simulink model "UPDATED_2"  (R2025a)
settings: Solver=VariableStepAuto  StartTime=0.0  StopTime=0  RelTol=1e-3
libraries: spsPWMGeneratorDCDCLib x8, spsSeriesRLCBranchLib x6, spsCurrentMeasurementLib x5, spsMosfetLib x4, spsVoltageMeasurementLib x3, eeStairGenerator x2, spsDCVoltageSourceLib x1, spsGroundLib x1, sps_lib x1
settings Model: Creator=KAILASH  LastModifiedBy=KAILASH

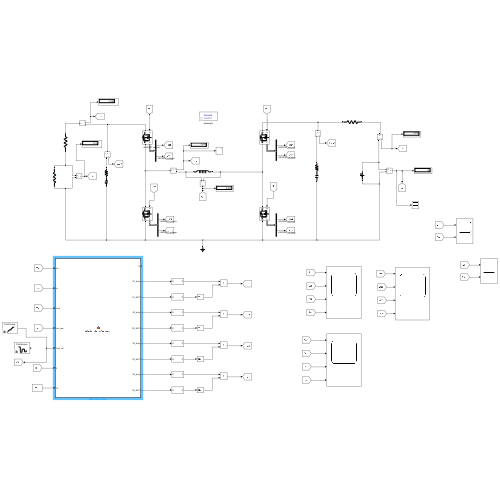
[thumbnail: Simulink's stored preview of the top-level diagram]
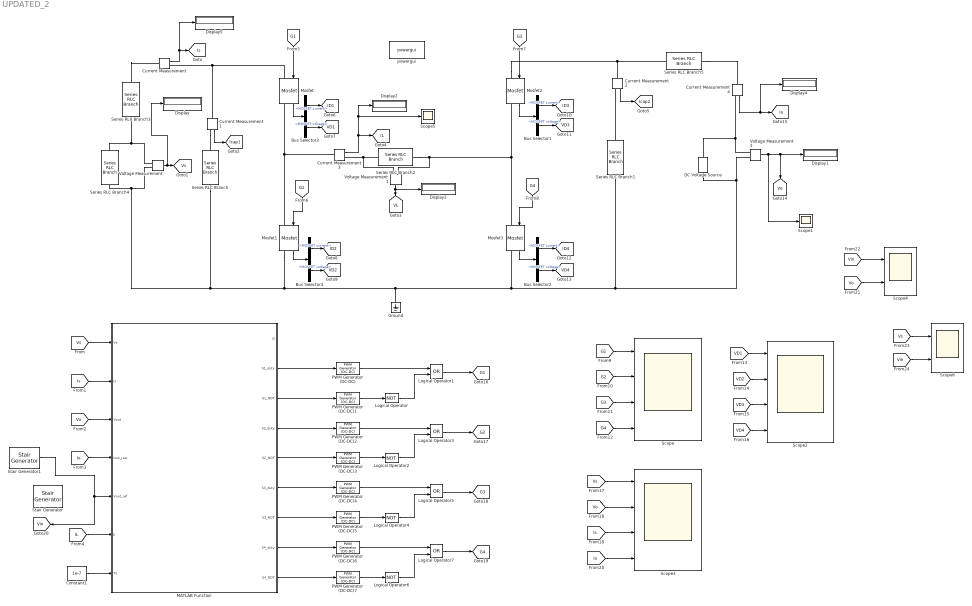
== system UPDATED_2 ==
  Bus Selector{1..4} (4 alike) : BusSelector  OutputSignals=MOSFET current,MOSFET voltage
  Constant1 : Constant  Value=1e-7
  Current Measurement{,1..4} (5 alike) : spsCurrentMeasurementLib/Current Measurement  PhasorSimulation=off  OutputType=Complex  PSBequivalent=0
  DC Voltage Source : spsDCVoltageSourceLib/DC Voltage Source  Amplitude=48  Measurements=Voltage
  Display{,1..5} (6 alike) : Display
  Ground : spsGroundLib/Ground  LConnTagsString=a
  Logical Operator{,2,4,6} (4 alike) : Logic  Operator=NOT  AllPortsSameDT=off  OutDataTypeStr=boolean
  Logical Operator{1,3,5,7} (4 alike) : Logic  Operator=OR  AllPortsSameDT=off  OutDataTypeStr=boolean
  MATLAB Function : MATLAB Function  TreatAsAtomicUnit=on
  Mosfet{,1..3} (4 alike) : spsMosfetLib/Mosfet  Ron=0.01  Lon=0  Rd=0.01  Vfd=0.8  IC=0  Rs=1e5  Cs=inf  Measurements=on
  PWM Generator (DC-DC){,1..7} (8 alike) : spsPWMGeneratorDCDCLib/PWM Generator (DC-DC)  Fsw=75e3  Ts=1e-7
  Scope : Scope  NumInputPorts=4
      settings: ActiveDisplayYMinimum=0.9  ActiveDisplayYMaximum=1.1
  Scope1 : Scope
      settings: ActiveDisplayYMinimum=-5.735151236633631  ActiveDisplayYMaximum=51.67637083167557
  Scope2 : Scope  NumInputPorts=4
      settings: ActiveDisplayYMinimum=-4.0101855999563254  ActiveDisplayYMaximum=36.044750018114769  DataLoggingVariableName=ScopeData2
  Scope3 : Scope  NumInputPorts=4
      settings: ActiveDisplayYMinimum=38  ActiveDisplayYMaximum=58  DataLoggingVariableName=ScopeData3
  Scope4 : Scope  NumInputPorts=2
      settings: ActiveDisplayYMinimum=-8.760106786096161  ActiveDisplayYMaximum=78.7511229762329  DataLoggingVariableName=ScopeData4
  Scope5 : Scope
      settings: ActiveDisplayYMinimum=-12.405117620742399  ActiveDisplayYMaximum=103.6893246645467  DataLoggingVariableName=ScopeData5
  Scope6 : Scope  NumInputPorts=2
      settings: ActiveDisplayYMinimum=-11.293274527726584  ActiveDisplayYMaximum=84.8994228584227  DataLoggingVariableName=ScopeData6
  Series RLC Branch : spsSeriesRLCBranchLib/Series RLC Branch  LConnTagsString=__new0  RConnTagsString=__new0  BranchType=RC  Resistance=0.001  Inductance=1e-3  SetiL0=off  InitialCurrent=0  Capacitance=488e-6  Setx0=off  InitialVoltage=48  Measurements=None
  Series RLC Branch1 : spsSeriesRLCBranchLib/Series RLC Branch  LConnTagsString=__new0  RConnTagsString=__new0  BranchType=RC  Resistance=0.01  Inductance=1e-3  SetiL0=off  InitialCurrent=0  Capacitance=488e-6  Setx0=off  InitialVoltage=36  Measurements=None
  Series RLC Branch2 : spsSeriesRLCBranchLib/Series RLC Branch  LConnTagsString=__new0  RConnTagsString=__new0  BranchType=L  Resistance=1  Inductance=200e-6  SetiL0=off  InitialCurrent=0  Capacitance=1e-6  Setx0=off  InitialVoltage=0  Measurements=None
  Series RLC Branch3 : spsSeriesRLCBranchLib/Series RLC Branch  LConnTagsString=__new0  RConnTagsString=__new0  BranchType=R  Resistance=1  Inductance=1e-3  SetiL0=off  InitialCurrent=0  Capacitance=1e-6  Setx0=off  InitialVoltage=0  Measurements=None
  Series RLC Branch4 : spsSeriesRLCBranchLib/Series RLC Branch  LConnTagsString=__new0  RConnTagsString=__new0  BranchType=R  Resistance=50  Inductance=1e-3  SetiL0=off  InitialCurrent=0  Capacitance=1e-6  Setx0=off  InitialVoltage=0  Measurements=None
  Series RLC Branch5 : spsSeriesRLCBranchLib/Series RLC Branch  LConnTagsString=__new0  RConnTagsString=__new0  BranchType=R  Resistance=1  Inductance=1e-3  SetiL0=off  InitialCurrent=0  Capacitance=1e-6  Setx0=off  InitialVoltage=0  Measurements=None
  Stair Generator : eeStairGenerator/Stair Generator  LabelModeActiveChoice=Continuous  TimeInput=[0.05 0.2 0.35 0.55 0.7]  AmplitudeInput=[90 6 55 12 36]  SampleTime=0  RepeatPattern=off  OutDataTypeStr=double
      settings: LibrarySourceBlock=ee_sl_lib/General Control/Stair Generator
  Stair Generator1 : eeStairGenerator/Stair Generator  LabelModeActiveChoice=Continuous  TimeInput=[0.05 0.2 0.35 0.55 0.7 0.85]  AmplitudeInput=[52 64 70 82 90 92]  SampleTime=0  RepeatPattern=off  OutDataTypeStr=double
      settings: LibrarySourceBlock=ee_sl_lib/General Control/Stair Generator
  Voltage Measurement : spsVoltageMeasurementLib/Voltage Measurement  PhasorSimulation=off  OutputType=Complex  PSBequivalent=0
  Voltage Measurement1 : spsVoltageMeasurementLib/Voltage Measurement  PhasorSimulation=off  OutputType=Complex  PSBequivalent=0
  Voltage Measurement2 : spsVoltageMeasurementLib/Voltage Measurement  PhasorSimulation=off  OutputType=Complex  PSBequivalent=0
  powergui : sps_lib/powergui  Priority=1  SimulationMode=Discrete  SampleTime=1e-7  frequency=60  Iterations=50  frequencyindice=0  Pbase=100e6  ErrMax=1e-4  UnitsV=kV  UnitsW=MW  buscounter=0  FunctionMessages=off  echomessages=off  EnableUseOfTLC=off  CurrentSourceSwitches=off  DisableSnubberDevices=off  DisableRonSwitches=off  DisableVfSwitches=off  DisplayEquations=off  AutomaticDiscreteSolvers=off  SolverType=Tustin/Backward Euler (TBE)  Interpol=off  ExternalGateDelay=off  methode=off  Ts=100  x0status=blocks  SPID=on  SwTol=0  HookPort=off  NonlinearTolerance=1e-4  nMaxIteration=100  ContinueOnMaxIteration=off  RestoreLinks=warning  ResistiveCurrentMeasurement=off  Frange=[0:2:500]  Ylog=off  Xlog=on  ShowGrid=off  save=off  variable=ZData  structure=0  ZoomFFT=off  StartTime=0.0  cycles=1  DisplayStyle=1  fundamental=60  FreqAxis=off  MaxFrequency=1000  frequencyindicesteady=1  RmsSteady=1  display=off
  tag scope: G1=global, G2=global, G3=global, G4=global, ID1=global, ID2=global, ID3=global, ID4=global, IL=global, Icap1=global, Icap2=global, Io=global, Is=global, VD1=global, VD2=global, VD3=global, VD4=global, VL=global, Vin=global, Vo=global, Vs=global
  wires:
  MATLAB Function/5(S2_NOT) -> PWM Generator (DC-DC)3/1
  Current Measurement1/1 -> [Icap1]
  Mosfet/1 -> Bus Selector3/1
  Bus Selector2/1 -> [ID4]  "<MOSFET current>"
  [G1] -> Scope/1
  MATLAB Function/7(S3_NOT) -> PWM Generator (DC-DC)5/1
  [Is] -> MATLAB Function/2(Is)
  MATLAB Function/8(S4_duty) -> PWM Generator (DC-DC)6/1
  [VD3] -> Scope2/3
  [Vo] -> Scope4/2
  PWM Generator (DC-DC)1/1 -> Logical Operator/1
  MATLAB Function/2(S1_duty) -> PWM Generator (DC-DC)/1
  PWM Generator (DC-DC)7/1 -> Logical Operator6/1
  Current Measurement3/1 -> [IL], Scope5/1, Display2/1
  Constant1/1 -> MATLAB Function/7(Ts)
  [Vo] -> MATLAB Function/3(Vout)
  Logical Operator7/1 -> [G4]
  Current Measurement/1 -> Display5/1, [Is]
  Mosfet1/1 -> Bus Selector4/1
  Logical Operator2/1 -> Logical Operator3/2
  [VD4] -> Scope2/4
  [G2] -> Mosfet1/1
  Logical Operator1/1 -> [G1]
  MATLAB Function/4(S2_duty) -> PWM Generator (DC-DC)2/1
  [G4] -> Scope/4
  MATLAB Function/3(S1_NOT) -> PWM Generator (DC-DC)1/1
  Voltage Measurement2/1 -> Scope1/1, [Vo], Display1/1
  PWM Generator (DC-DC)4/1 -> Logical Operator5/1
  Voltage Measurement/1 -> Display/1, [Vs]
  Bus Selector4/1 -> [ID2]  "<MOSFET current>"
  Logical Operator3/1 -> [G2]
  Mosfet2/1 -> Bus Selector1/1
  Bus Selector4/2 -> [VD2]  "<MOSFET voltage>"
  Logical Operator5/1 -> [G3]
  Stair Generator1/1 -> [Vin], MATLAB Function/5(Vout_ref)
  Current Measurement2/1 -> [Icap2]
  Current Measurement4/1 -> Display4/1, [Io]
  Logical Operator6/1 -> Logical Operator7/2
  [G1] -> Mosfet/1
  PWM Generator (DC-DC)2/1 -> Logical Operator3/1
  PWM Generator (DC-DC)/1 -> Logical Operator1/1
  PWM Generator (DC-DC)3/1 -> Logical Operator2/1
  Bus Selector3/1 -> [ID1]  "<MOSFET current>"
  [G2] -> Scope/2
  MATLAB Function/6(S3_duty) -> PWM Generator (DC-DC)4/1
  Voltage Measurement1/1 -> Display3/1, [VL]
  [Vs] -> Scope3/1
  [Io] -> Scope3/4
  [Vo] -> Scope3/2
  Bus Selector1/1 -> [ID3]  "<MOSFET current>"
  [Is] -> Scope3/3
  [IL] -> MATLAB Function/6(Il)
  Logical Operator4/1 -> Logical Operator5/2
  Logical Operator/1 -> Logical Operator1/2
  [VD1] -> Scope2/1
  [Io] -> MATLAB Function/4(Iout_raw)
  [Vin] -> Scope4/1
  [Vs] -> MATLAB Function/1(Vs)
  [G3] -> Mosfet2/1
  Bus Selector1/2 -> [VD3]  "<MOSFET voltage>"
  MATLAB Function/9(S4_NOT) -> PWM Generator (DC-DC)7/1
  Mosfet3/1 -> Bus Selector2/1
  PWM Generator (DC-DC)5/1 -> Logical Operator4/1
  Bus Selector3/2 -> [VD1]  "<MOSFET voltage>"
  [G3] -> Scope/3
  [VD2] -> Scope2/2
  Bus Selector2/2 -> [VD4]  "<MOSFET voltage>"
  [G4] -> Mosfet3/1
  PWM Generator (DC-DC)6/1 -> Logical Operator7/1
  [Vs] -> Scope6/1
  [Vin] -> Scope6/2
  connections:
  Mosfet3/RConn1 -- DC Voltage Source/LConn1 -- Voltage Measurement2/LConn2 -- Series RLC Branch1/RConn1 -- Ground/LConn1 -- Mosfet1/RConn1 -- Series RLC Branch/RConn1 -- Series RLC Branch4/RConn1 -- Voltage Measurement/LConn2
  Voltage Measurement1/LConn1 -- Current Measurement3/RConn1 -- Series RLC Branch2/LConn1
  Current Measurement3/LConn1 -- Mosfet/RConn1 -- Mosfet1/LConn1
  Mosfet2/LConn1 -- Series RLC Branch5/LConn1 -- Current Measurement2/LConn1
  Voltage Measurement2/LConn1 -- DC Voltage Source/RConn1 -- Current Measurement4/RConn1
  Voltage Measurement/LConn1 -- Series RLC Branch4/LConn1 -- Series RLC Branch3/LConn1
  Current Measurement1/LConn1 -- Current Measurement/RConn1 -- Mosfet/LConn1
  Voltage Measurement1/LConn2 -- Series RLC Branch2/RConn1 -- Mosfet2/RConn1 -- Mosfet3/LConn1
  Current Measurement1/RConn1 -- Series RLC Branch/LConn1
  Series RLC Branch3/RConn1 -- Current Measurement/LConn1
  Series RLC Branch5/RConn1 -- Current Measurement4/LConn1
  Series RLC Branch1/LConn1 -- Current Measurement2/RConn1

== matlab function UPDATED_2/MATLAB Function ==
  data: Vs input; Is input; D output; Vout input; Iout_raw input; Vout_ref input; Il input; Ts input; S1_duty output; S1_NOT output; S2_duty output; S2_NOT output; S3_duty output; S3_NOT output; S4_duty output; S4_NOT output
function [D, S1_duty, S1_NOT, S2_duty, S2_NOT, S3_duty, S3_NOT, S4_duty, S4_NOT] = biDirBuckBoostController(Vs, Is, Vout, Iout_raw, Vout_ref, Il, Ts)
% Streamlined Bidirectional Controller
% Features: Smart Auto-Startup, Hybrid Transition Logic, Perfect Discharge Mirror

%% ===================== 1. GLOBAL LIMITS & SETTINGS =====================
D_MAX = 1.0;
D_MIN = 0.0;
V_HYST = 3.0;
I_DEADBAND = 0.1;
I_TARGET_MAX = 50.0;
I_TARGET_MIN = -50.0;

%% ===================== 2. PERSISTENT MEMORY (STATE VARIABLES) =====================
persistent is_charging_state
persistent v_int_chg i_int_chg
persistent v_int_dis i_int_dis R_est_prev
persistent prev_Vout_ref was_falling
persistent prev_Vref_led was_falling_dis 

% --- STATIC INITIALIZATION ---
if isempty(v_int_chg), v_int_chg = 0.0; end
if isempty(i_int_chg), i_int_chg = 0.0; end
if isempty(v_int_dis), v_int_dis = 0; end
if isempty(i_int_dis), i_int_dis = 0; end
if isempty(R_est_prev), R_est_prev = 3.0;end
if isempty(prev_Vout_ref), prev_Vout_ref = 0.0; end
if isempty(was_falling), was_falling = false; end
if isempty(prev_Vref_led), prev_Vref_led = 0.0; end
if isempty(was_falling_dis), was_falling_dis = false; end

% --- SMART AUTO-STARTUP (Fixes the Mode-Switching Spike at t=0) ---
if isempty(is_charging_state)
    if Vout > Vs + 5.0
        is_charging_state = false; % Battery is on Vout -> Start in Discharge!
    else
        is_charging_state = true;  % Battery is on Vs -> Start in Charge!
    end
end

%% ===================== 3. AUTO-MODE DETECTION =====================
if is_charging_state == true
    if Il < -I_DEADBAND
        is_charging_state = false;
    end
else
    if Il > I_DEADBAND
        is_charging_state = true;
    end
end
is_charging = is_charging_state;

%% ===================== 4. MODE 1: CHARGE CONTROL (Vs -> Vout) =====================
if is_charging
    % --- TOPOLOGY DETECTION ---
    if Vs > Vout_ref + V_HYST
        current_topology = 1; % BUCK
    elseif Vs < Vout_ref - V_HYST
        current_topology = 2; % BOOST
    else
        current_topology = 3; % BUCK-BOOST
    end
    
    % --- LOGIC 1: THE DEPARTURE "MUSCLE" (For Stepping UP) ---
    if abs(Vout_ref - prev_Vout_ref) > 1.0
        if Vout_ref < prev_Vout_ref
            was_falling = true; % Arm the catch for the down-step parachute
        else
            % Stepping UP:
            % ONLY reset if we are crossing from BUCK/OFF into BOOST.
            % If we are already inside the BOOST region, DO NOT RESET!
            if current_topology == 2 && prev_Vout_ref <= Vs + V_HYST
                i_int_chg = 0.0;
                v_int_chg = 1.0;
            end
        end
    end
    prev_Vout_ref = Vout_ref;
    v_err = Vout_ref - Vout;
    
    % --- LOGIC 2: THE ARRIVAL "CATCH" (For Stepping DOWN) ---
    if was_falling && v_err >= 0
        % Voltage landed on the target! Deploy the parachute math.
        v_int_chg = Iout_raw;
        if current_topology == 1 % BUCK
            i_int_chg = Vout_ref / Vs; % Inject exact duty cycle needed
        else % BOOST
            i_int_chg = max(0, 1 - (Vs / max(Vout_ref, 1e-3)));
        end
        was_falling = false; % Disarm catch
    end
    
    % --- UNIFIED CHARGE GAINS ---
    Kp_v = 0.02; Ki_v = 1.0;
    Kp_i = 0.10; Ki_i = 40.0;
    
    % --- Outer Voltage Loop ---
    v_P = Kp_v * v_err;
    I_unsat = v_P + v_int_chg;
    I_target = min(max(I_unsat, I_TARGET_MIN), I_TARGET_MAX);
    v_I_step = Ki_v * v_err * Ts;
    
    if (I_unsat > I_TARGET_MAX && v_err > 0) || (I_unsat < I_TARGET_MIN && v_err < 0)
        % Clamped
    else
        v_int_chg = v_int_chg + v_I_step;
    end
    
    % --- Inner Current Loop ---
    i_err = I_target - Iout_raw;
    i_P = Kp_i * i_err;
    D_unsat = i_P + i_int_chg;
    D = min(max(D_unsat, D_MIN), D_MAX);
    i_I_step = Ki_i * i_err * Ts;
    
    if (D_unsat > D_MAX && i_err > 0) || (D_unsat < D_MIN && i_err < 0)
        % Clamped
    else
        i_int_chg = i_int_chg + i_I_step;
    end
    
    % --- Dynamic Charge Switch Mapping ---
    if current_topology == 1 % BUCK
        S1_duty = D; S1_NOT = 1.0; S2_duty = 0.0; S2_NOT = D;
        S3_duty = 1.0; S3_NOT = 1.0; S4_duty = 0.0; S4_NOT = 1.0;
    elseif current_topology == 2 % BOOST
        S1_duty = 1.0; S1_NOT = 1.0; S2_duty = 0.0; S2_NOT = 1.0;
        S3_duty = 0.0; S3_NOT = D; S4_duty = D; S4_NOT = 1.0;
    else % TRANSITION
        S1_duty = D; S1_NOT = 1.0; S2_duty = 0.0; S2_NOT = D;
        S3_duty = 0.0; S3_NOT = D; S4_duty = D; S4_NOT = 1.0;
    end
    return;
    
%% ===================== 5. MODE 2: DISCHARGE CONTROL (Vout -> Vs) =====================
else
    % Discharge targets (Now perfectly tracking the stair generator)
    Vref_led = Vout_ref;

    % Reverse the measurement perspectives
    I_load_raw = -Is;
    V_load = Vs;
    V_batt = Vout;

    % --- REVERSE TOPOLOGY DETECTION ---
    if V_batt > Vref_led + V_HYST
        current_topology_dis = 1; % REVERSE BUCK
    elseif V_batt < Vref_led - V_HYST
        current_topology_dis = 2; % REVERSE BOOST
    else
        current_topology_dis = 3; % REVERSE BUCK-BOOST
    end

    % --- LOGIC 1: THE DEPARTURE "MUSCLE" (For Stepping UP Reverse Voltage) ---
    if abs(Vref_led - prev_Vref_led) > 1.0
        if Vref_led < prev_Vref_led
            was_falling_dis = true; % Arm the catch for the down-step parachute
        else
            % Stepping UP: ONLY reset if crossing into Reverse Boost.
            if current_topology_dis == 2 && prev_Vref_led <= V_batt + V_HYST
                i_int_dis = 0.0;
                v_int_dis = 1.0;
            end
        end
    end
    prev_Vref_led = Vref_led;
    v_err = Vref_led - V_load;

    % --- LOGIC 2: THE ARRIVAL "CATCH" (For Stepping DOWN Reverse Voltage) ---
    if was_falling_dis && v_err >= 0
        % Voltage landed on target!
        v_int_dis = I_load_raw;
        if current_topology_dis == 1 % REVERSE BUCK
            i_int_dis = Vref_led / V_batt;
        else % REVERSE BOOST
            i_int_dis = max(0, 1 - (V_batt / max(Vref_led, 1e-3)));
        end
        was_falling_dis = false;
    end

    % --- DISCHARGE GAINS (Identical Mirror of Charge) ---
    Kp_v_dis = 0.02; Ki_v_dis = 1.0;
    Kp_i_dis = 0.10; Ki_i_dis = 40.0;

    % --- Outer Voltage Loop (Reverse) ---
    v_P = Kp_v_dis * v_err;
    I_unsat = v_P + v_int_dis;
    I_target = min(max(I_unsat, I_TARGET_MIN), I_TARGET_MAX);
    v_I_step = Ki_v_dis * v_err * Ts;
    if (I_unsat > I_TARGET_MAX && v_err > 0) || (I_unsat < I_TARGET_MIN && v_err < 0)
        % Clamped
    else
        v_int_dis = v_int_dis + v_I_step;
    end

    % --- Inner Current Loop (Reverse) ---
    i_err = I_target - I_load_raw;
    i_P = Kp_i_dis * i_err;
    D_unsat = i_P + i_int_dis;
    D = min(max(D_unsat, D_MIN), D_MAX);
    i_I_step = Ki_i_dis * i_err * Ts;
    if (D_unsat > D_MAX && i_err > 0) || (D_unsat < D_MIN && i_err < 0)
        % Clamped
    else
        i_int_dis = i_int_dis + i_I_step;
    end

    % --- Dynamic Reverse Switch Mapping ---
    if current_topology_dis == 1 % REVERSE BUCK
        S1_duty = 1.0; S1_NOT = 1.0; S2_duty = 0.0; S2_NOT = 1.0;
        S3_duty = D;   S3_NOT = 1.0; S4_duty = 0.0; S4_NOT = D;
    elseif current_topology_dis == 2 % REVERSE BOOST
        S1_duty = 0.0; S1_NOT = D;   S2_duty = D;   S2_NOT = 1.0;
        S3_duty = 1.0; S3_NOT = 1.0; S4_duty = 0.0; S4_NOT = 1.0;
    else % TRANSITION
        S1_duty = 0.0; S1_NOT = D;   S2_duty = D;   S2_NOT = 1.0;
        S3_duty = D;   S3_NOT = 1.0; S4_duty = 0.0; S4_NOT = D;
    end
    return;
end
end
